simulink library "carnot"  (R2018b)
settings: Solver=VariableStepAuto  StartTime=0.0  StopTime=10.0  RelTol=1e-3
undefined symbols (not defined in the file or in its folder): A, A_earth, acol, Acol, ActPower1, ActPower2, ActPower3, Ad, Ad0, Ar, Au, Au0, Azimuth_Angle, B, Bd, Bd0, Br, Bu, Bu0, C, c1, c2, c3, c33, c4, c5, c6, CarnotCallbacks_Density, CarnotCallbacks_Enthalpy, CarnotCallbacks_Enthalpy2Temperature, CarnotCallbacks_Entropy, CarnotCallbacks_Evaporation_Enthalpy, CarnotCallbacks_GlobalMessageLevel, CarnotCallbacks_Grashof, CarnotCallbacks_Heat_Capacity, CarnotCallbacks_Kinematic_Viscosity, CarnotCallbacks_PMV_PPD, CarnotCallbacks_Prandtl, CarnotCallbacks_Saturation_Property, CarnotCallbacks_Saturation_Temperature, CarnotCallbacks_Saturation_Value_Water, CarnotCallbacks_Specific_Volume, CarnotCallbacks_Thermal_Conductivity, CarnotCallbacks_Vapour_Content, CarnotCallbacks_Vapour_Pressure, Cd, Cdl, Cr, Cu, Davies, Dd, DE_TRY2010_04_averageYear, delta_grd, density, DiameterLastPiece, dl, DPConstant, DPLinear, DPQuadratic, Dr ... (+59)
libraries: $bdroot x429, simulink x36, simulink_extras x12
(part 5 of 22)

== system carnot/Basic/Material_Properties ==
  AIV_WetBulbTemperature : Subsystem  mask(AIV to wet bulb temperature and relative humidity){}
      mask help:
      | Calculate  - the relative humidity of air (rH)
      |                  - and the wet bulb temperature of air (WBT)
      | from          - dry bulb air temperature (DBT)
      |                  - and mass of water per mass of air (x)
      | in AIV vector.
      |
      | DBT        [degree centigrade]
      | p              [Pa]
      | x              kg water / kg air
      |
      | rel_hum   [percent]
      | WBT       [degree centigrade] -> T_WBT is valid for T [-6..40°C]
      mask Help: web(fullfile(path_carnot('help'),'AIV_Wet_BulbTemperature.html'),'-helpbrowser')
  Density : Subsystem  LoadFcn=CarnotCallbacks_Density('LoadFcn');  InitFcn=load('THB.mat');  VariantControl=CarlibClassic  mask(density){INPUTARGUMENTS=state variables (classic), DEBUGLEVEL=DEBUGLEVEL, MAXTOTALWARNINGS=inf, MAXCONSECUTIVEWARNINGS=inf, WRITETOFILE=0, FILENAME='errors.txt'}
      mask prompts: INPUTARGUMENTS "Input arguments"; DEBUGLEVEL "Debug level"; MAXTOTALWARNINGS "maximum number of total warning"; MAXCONSECUTIVEWARNINGS "maximum number of consecutive warnings"; WRITETOFILE "write messages to file"; FILENAME "filename for error messages"
      mask help:
      | Calculates the fluid density  [kg/m³]. Calls the function "density" in the CARNOT library "carlib".
      | You may use the block "GlobalMessageLevel" in the Toolbox to handle the debugging messages.
      | FluidType        Remarks
      | 1: water          fluid mix is vapourcontent in the 2-phase region
      | 2: air              fluid mix is (kg water) / (kg dry air)
      | 3: cotton oil       -
      | 4: silicone oil     -
      | 5: water-glycol   fluid mix is volume partition [0..1] of propylen glycol
      | 6: Tyfocor LS     function only available in liquid phase
      | 7: Water Constant = 998.21 kg/m³ (water at 20°C)
      | 8: Air Constant   = 1.118 kg/m³ (air at 20°C)
      mask init:
      | %Inports
      | CarnotCallbacks_Density('CreateInports');
      | 
      | %global debug level
      | [DEBUGLEVEL, MAXTOTALWARNINGS, MAXCONSECUTIVEWARNINGS, WRITETOFILE, FILENAME] = CarnotCallbacks_Density('CheckDebugLevels', DEBUGLEVEL, MAXTOTALWARNINGS, MAXCONSECUTIVEWARNINGS, WRITETOFILE, FILENAME);
      mask Help: web(fullfile(path_carnot('help'),'density_mdl.html'),'-helpbrowser')
      mask TypeOptions INPUTARGUMENTS: state variables (classic) | THB | THV
      mask Callback INPUTARGUMENTS: CarnotCallbacks_Density('MaskVisibilities');
      mask TypeOptions DEBUGLEVEL: DEBUGLEVEL | INFOLEVEL | WARNINGLEVEL | ERRORLEVEL | FATALLEVEL | NOLEVEL
      mask DialogControl ParameterTabVar0 Prompt: Parameters
      mask DialogControl ParameterTabVar01 Prompt: Debugging
  Enthalpy : Subsystem  LoadFcn=CarnotCallbacks_Enthalpy('LoadFcn');  InitFcn=load('THB.mat');  VariantControl=CarlibClassic  mask(enthalpy){INPUTARGUMENTS=state variables (classic), DEBUGLEVEL=WARNINGLEVEL, MAXTOTALMESSAGES=inf, MAXCONSECUTIVEMESSAGES=inf, WRITETOFILE=0, FILENAME='errors.txt'}
      mask prompts: INPUTARGUMENTS "Input arguments"; DEBUGLEVEL "Debug level"; MAXTOTALMESSAGES "maximum number of total warning"; MAXCONSECUTIVEMESSAGES "maximum number of consecutive warnings"; WRITETOFILE "write messages to file"; FILENAME "filename for error messages"
      mask help:
      | Calculates the fluid specific enthalpy  [J/kg].
      | Calls the CARNOT library "carlib".
      | WORKS FOR WATER AND DRY AIR! Enthalpy for other fluids is cp*T.
      | FluidType        Remarks
      | 1: water          fluid mix is vapourcontent in the 2-phase region
      | 2: air              fluid mix is (kg water) / (kg dry air)
      | 3: cotton oil       -
      | 4: silicone oil     -
      | 5: water-glycol   fluid mix is volume partition [0..1] of propylen glycol
      | 6: Tyfocor LS     function only available in liquid phase
      | 7: Water Constant = 0.0 J/kg (water at 20°C)
      | 8: Air Constant   = 0.0 J/kg (air at 20°C)
      mask init:
      | %Inports
      | CarnotCallbacks_Enthalpy('CreateInports');
      | 
      | %global debug level
      | [DEBUGLEVEL, MAXTOTALMESSAGES, MAXCONSECUTIVEMESSAGES, WRITETOFILE, FILENAME] = CarnotCallbacks_Enthalpy('CheckDebugLevels', DEBUGLEVEL, MAXTOTALMESSAGES, MAXCONSECUTIVEMESSAGES, WRITETOFILE, FILENAME);
      mask Help: web(fullfile(path_carnot('help'),'enthalpy_mdl.html'),'-helpbrowser')
      mask TypeOptions INPUTARGUMENTS: state variables (classic) | THB | THV
      mask Callback INPUTARGUMENTS: CarnotCallbacks_Enthalpy('MaskVisibilities');
      mask TypeOptions DEBUGLEVEL: DEBUGLEVEL | INFOLEVEL | WARNINGLEVEL | ERRORLEVEL | FATALLEVEL | NOLEVEL
      mask DialogControl ParameterTabVar0 Prompt: Parameters
      mask DialogControl ParameterTabVar01 Prompt: Debugging
  Enthalpy2Temperature : Subsystem  LoadFcn=CarnotCallbacks_Enthalpy2Temperature('LoadFcn');  VariantControl=CarlibClassic  mask(Enthalpy to Temperature){DEBUGLEVEL=WARNINGLEVEL, MAXTOTALMESSAGES=inf, MAXCONSECUTIVEMESSAGES=inf, WRITETOFILE=0, FILENAME='errors.txt'}
      mask prompts: DEBUGLEVEL "Debug level"; MAXTOTALMESSAGES "maximum number of total warning"; MAXCONSECUTIVEMESSAGES "maximum number of consecutive warnings"; WRITETOFILE "write messages to file"; FILENAME "filename for error messages"
      mask help:
      | Calculates the temperature  [°C] from the fluid Enthalpy [J/kg].
      | Enthalpy may be a scalar or a vector. All other inputs must be scalar.
      | FluidType        Remarks
      | 1: water          fluid mix is vapourcontent in the 2-phase region
      | 2: air              fluid mix is (kg water) / (kg dry air)
      | 3: cotton oil       -
      | 4: silicone oil     -
      | 5: water-glycol   fluid mix is volume partition [0..1] of propylen glycol
      | 6: Tyfocor LS     function only available in liquid phase
      | 7: Water Constant - function not defined
      | 8: Air Constant - function not defined
      mask init:
      | %global debug level
      | [DEBUGLEVEL, MAXTOTALMESSAGES, MAXCONSECUTIVEMESSAGES, WRITETOFILE, FILENAME] = CarnotCallbacks_Enthalpy2Temperature('CheckDebugLevels', DEBUGLEVEL, MAXTOTALMESSAGES, MAXCONSECUTIVEMESSAGES, WRITETOFILE, FILENAME);
      mask Help: web(fullfile(path_carnot('help'),'enthalpy2temperature_mdl.html'),'-helpbrowser')
      mask TypeOptions DEBUGLEVEL: DEBUGLEVEL | INFOLEVEL | WARNINGLEVEL | ERRORLEVEL | FATALLEVEL | NOLEVEL
      mask DialogControl ParameterTabVar0 Prompt: Debugging
  Entropy : Subsystem  LoadFcn=CarnotCallbacks_Entropy('LoadFcn');  InitFcn=load('THB.mat');  VariantControl=CarlibClassic  mask(entropy){INPUTARGUMENTS=state variables (classic), DEBUGLEVEL=WARNINGLEVEL, MAXTOTALMESSAGES=inf, MAXCONSECUTIVEMESSAGES=inf, WRITETOFILE=0, FILENAME='errors.txt'}
      mask prompts: INPUTARGUMENTS "Input arguments"; DEBUGLEVEL "Debug level"; MAXTOTALMESSAGES "maximum number of total warning"; MAXCONSECUTIVEMESSAGES "maximum number of consecutive warnings"; WRITETOFILE "write messages to file"; FILENAME "filename for error messages"
      mask help:
      | The block calculates the entropy  [J/kgK] of the fluid.
      | The block calls the function "entropy" in the CARNOT library "carlib".
      | FluidType        Remarks
      | 1: water          fluid mix is vapourcontent in the 2-phase region
      | 2: air              fluid mix is (kg water) / (kg dry air)
      | 3: cotton oil       -
      | 4: silicone oil     -
      | 5: water-glycol   fluid mix is volume partition [0..1] of propylen glycol
      | 6: Tyfocor LS     function only available in liquid phase
      | 7: Water Constant = 0.0 J/K/kg
      | 8: Air Constant   = 0.0 J/K/kg
      mask init:
      | %Inports
      | CarnotCallbacks_Entropy('CreateInports');
      | 
      | %global debug level
      | [DEBUGLEVEL, MAXTOTALMESSAGES, MAXCONSECUTIVEMESSAGES, WRITETOFILE, FILENAME] = CarnotCallbacks_Entropy('CheckDebugLevels', DEBUGLEVEL, MAXTOTALMESSAGES, MAXCONSECUTIVEMESSAGES, WRITETOFILE, FILENAME);
      mask Help: web(fullfile(path_carnot('help'),'entropy.html'),'-helpbrowser')
      mask TypeOptions INPUTARGUMENTS: state variables (classic) | THB | THV
      mask Callback INPUTARGUMENTS: CarnotCallbacks_Entropy('MaskVisibilities');
      mask TypeOptions DEBUGLEVEL: DEBUGLEVEL | INFOLEVEL | WARNINGLEVEL | ERRORLEVEL | FATALLEVEL | NOLEVEL
      mask DialogControl ParameterTabVar0 Prompt: Parameters
      mask DialogControl ParameterTabVar01 Prompt: Debugging
  Evaporation_Enthalpy : Subsystem  LoadFcn=CarnotCallbacks_Evaporation_Enthalpy('LoadFcn');  InitFcn=load('THB.mat');  VariantControl=CarlibClassic  mask(entropy){INPUTARGUMENTS=state variables (classic), DEBUGLEVEL=WARNINGLEVEL, MAXTOTALMESSAGES=inf, MAXCONSECUTIVEMESSAGES=inf, WRITETOFILE=0, FILENAME='errors.txt'}
      mask prompts: INPUTARGUMENTS "Input arguments"; DEBUGLEVEL "Debug level"; MAXTOTALMESSAGES "maximum number of total warning"; MAXCONSECUTIVEMESSAGES "maximum number of consecutive warnings"; WRITETOFILE "write messages to file"; FILENAME "filename for error messages"
      mask help:
      | The block calculates the evaporation enthalpy [J/kgK] of water.
      | The block uses the material properties functions in carlib.
      | FluidType  material           remarks on fluid mix
      | 1           water              vapourcontent in the 2-phase region
      | all others: function not defined
      mask init:
      | %Inports
      | CarnotCallbacks_Evaporation_Enthalpy('CreateInports');
      | 
      | %global debug level
      | [DEBUGLEVEL, MAXTOTALMESSAGES, MAXCONSECUTIVEMESSAGES, WRITETOFILE, FILENAME] = CarnotCallbacks_Evaporation_Enthalpy('CheckDebugLevels', DEBUGLEVEL, MAXTOTALMESSAGES, MAXCONSECUTIVEMESSAGES, WRITETOFILE, FILENAME);
      mask Help: web(fullfile(path_carnot('help'),'evaporation_enthalpy_mdl.html'),'-helpbrowser')
      mask TypeOptions INPUTARGUMENTS: state variables (classic) | THB | THV
      mask Callback INPUTARGUMENTS: CarnotCallbacks_Evaporation_Enthalpy('MaskVisibilities');
      mask TypeOptions DEBUGLEVEL: DEBUGLEVEL | INFOLEVEL | WARNINGLEVEL | ERRORLEVEL | FATALLEVEL | NOLEVEL
      mask DialogControl ParameterTabVar0 Prompt: Parameters
      mask DialogControl ParameterTabVar01 Prompt: Debugging
  Heat_Capacity : Subsystem  LoadFcn=CarnotCallbacks_Heat_Capacity('LoadFcn');  InitFcn=load('THB.mat');  VariantControl=CarlibClassic  mask(heat capacity){INPUTARGUMENTS=state variables (classic), DEBUGLEVEL=DEBUGLEVEL, MAXTOTALWARNINGS=inf, MAXCONSECUTIVEWARNINGS=inf, WRITETOFILE=0, FILENAME='errors.txt'}
      mask prompts: INPUTARGUMENTS "Input arguments"; DEBUGLEVEL "Debug level"; MAXTOTALWARNINGS "maximum number of total warning"; MAXCONSECUTIVEWARNINGS "maximum number of consecutive warnings"; WRITETOFILE "write messages to file"; FILENAME "filename for error messages"
      mask help:
      | Calculates the  heat_capacity of fluids [J/(kg*K)]. Calls calls the function "heat_capacity" in the CARNOT library "carlib".
      | You may use the block "GlobalMessageLevel" in the Toolbox to handle the debugging messages.
      | FluidType        Remarks
      | 1: water          fluid mix is vapourcontent in the 2-phase region
      | 2: air              fluid mix is (kg water) / (kg dry air)
      | 3: cotton oil       -
      | 4: silicone oil     -
      | 5: water-glycol   fluid mix is volume partition [0..1] of propylen glycol
      | 6: Tyfocor LS     function only available in liquid phase
      | 7: Water Constant = 4181.0 J/kg/K (water at 20°C)
      | 8: Air Constant   = 1007.0 J/kg/K (air at 20°C)
      mask init:
      | %Inports
      | CarnotCallbacks_Heat_Capacity('CreateInports');
      | 
      | %global debug level
      | [DEBUGLEVEL, MAXTOTALWARNINGS, MAXCONSECUTIVEWARNINGS, WRITETOFILE, FILENAME] = CarnotCallbacks_Heat_Capacity('CheckDebugLevels', DEBUGLEVEL, MAXTOTALWARNINGS, MAXCONSECUTIVEWARNINGS, WRITETOFILE, FILENAME);
      mask Help: web(fullfile(path_carnot('help'),'heat_capacity_mdl.html'),'-helpbrowser')
      mask TypeOptions INPUTARGUMENTS: state variables (classic) | THB | THV
      mask Callback INPUTARGUMENTS: CarnotCallbacks_Heat_Capacity('MaskVisibilities');
      mask TypeOptions DEBUGLEVEL: DEBUGLEVEL | INFOLEVEL | WARNINGLEVEL | ERRORLEVEL | FATALLEVEL | NOLEVEL
      mask DialogControl ParameterTabVar0 Prompt: Parameters
      mask DialogControl ParameterTabVar01 Prompt: Debugging
  Input_Air : Subsystem  mask(Input_Air){T=20, p=1e5, x=0.005}
      mask prompts: T "temperature (scalar or vector) [°C]"; p "pressure [Pa]"; x "absolute humidity of moist air [kg water/kg dry air]"
      mask help:
      | Input block for the material "Air"
      |
      | The relevant inputs for the calculation of the block can be specified as parameter in the mask
      mask Help: web(fullfile(path_carnot('help'),'input_material.html'),'-helpbrowser')
  Input_Cotton_Oil : Subsystem  mask(Input_Cotton_Oil){T=20, p=1e5}
      mask prompts: T "temperature (scalar or vector) [°C]"; p "pressure [Pa]"
      mask help: Input block for the material "Cotton Oil". The relevant inputs for the calculation of the block can be specified as parameter in the mask
      mask Help: web(fullfile(path_carnot('help'),'input_material.html'),'-helpbrowser')
  Input_Fluid : Subsystem  mask(Input_Fluid){fluid=Water, T=[10:10:50], p=1e5, x=0.005}
      mask prompts: fluid "Fluid type"; T "temperature (scalar or vector) [°C]"; p "pressure [Pa]"; x "Fluid Mix"
      mask help:
      | FLUID            FLUID MIX
      | water          vapourcontent in the 2-phase region
      | air               (kg water) / (kg dry air)
      | cotton oil       -
      | silicone oil     -
      | water-glycol   volume partition [0..1] of propylen glycol
      mask Help: web(fullfile(path_carnot('help'),'input_material.html'),'-helpbrowser')
      mask TypeOptions fluid: Water | Air | Cotton Oil | Silicone Oil | Water-Glycol Mix | Tyfocor LS | Water (Constant 20°C) | Air (dry+ constant 20°C)
  Input_Silicon_Oil : Subsystem  mask(Input_Silicon_Oil){T=20, p=1e5}
      mask prompts: T "temperature (scalar or vector) [°C]"; p "pressure [Pa]"
      mask help: Input block for the material "Silicon_Oil". The relevant inputs for the calculation of the block can be specified as parameter in the mask
      mask Help: web(fullfile(path_carnot('help'),'input_material.html'),'-helpbrowser')
  Input_Tyfocor_LS : Subsystem  mask(Input_Tyfocor_LS){T=20, p=1e5}
      mask prompts: T "temperature (scalar or vector) [°C]"; p "pressure [Pa]"
      mask help:
      | Input block for the material "Tyfocor_LS". The relevant inputs for the calculation of the block can be specified as parameter in the mask.
      | Tyfocor is a registered trademark of Tyforop Chemie, Hamburg (Germany).
      mask Help: web(fullfile(path_carnot('help'),'input_material.html'),'-helpbrowser')
  Input_Water : Subsystem  mask(Input_Water){T=20, p=2e6, xd=0}
      mask prompts: T "temperature (scalar or vector) [°C]"; p "pressure [Pa]"; xd "vapour content of the water [0..1]"
      mask help:
      | Input block for the material "Water"
      |
      | The relevant inputs for the calculation of the block can be specified as parameter in the mask
      mask Help: web(fullfile(path_carnot('help'),'input_material.html'),'-helpbrowser')
  Input_Water_Glycol : Subsystem  mask(input_water_glycol){T=20, p=1e5, g=0.4}
      mask prompts: T "temperature (scalar or vector) [°C]"; p "pressure [Pa]"; g "volume content of glycol [0..1]"
      mask help: Sets all values for the water - propylen-glycol mixtures.
      mask Help: web(fullfile(path_carnot('help'),'input_material.html'),'-helpbrowser')
  Kinematic_Viscosity : Subsystem  LoadFcn=CarnotCallbacks_Kinematic_Viscosity('LoadFcn');  InitFcn=load('THB.mat');  VariantControl=CarlibClassic  mask(kinematic viscosity){INPUTARGUMENTS=state variables (classic), DEBUGLEVEL=WARNINGLEVEL, MAXTOTALMESSAGES=inf, MAXCONSECUTIVEMESSAGES=inf, WRITETOFILE=0, FILENAME='errors.txt'}
      mask prompts: INPUTARGUMENTS "Input arguments"; DEBUGLEVEL "Debug level"; MAXTOTALMESSAGES "maximum number of total warning"; MAXCONSECUTIVEMESSAGES "maximum number of consecutive warnings"; WRITETOFILE "write messages to file"; FILENAME "filename for error messages"
      mask help:
      | Calculates the kinematic viscosity of fluids [m²/s].
      | Calls the function "viscosity" in the CARNOT library "carlib".
      | FluidType        Remarks
      | 1: water          fluid mix is vapourcontent in the 2-phase region
      | 2: air              fluid mix is (kg water) / (kg dry air)
      | 3: cotton oil       -
      | 4: silicone oil     -
      | 5: water-glycol   fluid mix is volume partition [0..1] of propylen glycol
      | 6: Tyfocor LS     function only available in liquid phase
      | 7: Water Constant = 1.004e-6 m²/s (water at 20°C)
      | 8: Air Constant   = 15.35e-6 m²/s (air at 20°C)
      mask init:
      | %Inports
      | CarnotCallbacks_Kinematic_Viscosity('CreateInports');
      | 
      | %global debug level
      | [DEBUGLEVEL, MAXTOTALMESSAGES, MAXCONSECUTIVEMESSAGES, WRITETOFILE, FILENAME] = CarnotCallbacks_Kinematic_Viscosity('CheckDebugLevels', DEBUGLEVEL, MAXTOTALMESSAGES, MAXCONSECUTIVEMESSAGES, WRITETOFILE, FILENAME);
      mask Help: web(fullfile(path_carnot('help'),'kinematic_viscosity_mdl.html'),'-helpbrowser')
      mask TypeOptions INPUTARGUMENTS: state variables (classic) | THB | THV
      mask Callback INPUTARGUMENTS: CarnotCallbacks_Kinematic_Viscosity('MaskVisibilities');
      mask TypeOptions DEBUGLEVEL: DEBUGLEVEL | INFOLEVEL | WARNINGLEVEL | ERRORLEVEL | FATALLEVEL | NOLEVEL
      mask DialogControl ParameterTabVar0 Prompt: Parameters
      mask DialogControl ParameterTabVar01 Prompt: Debugging
  PhaseCheck : Subsystem  mask(phasecheck){}
      mask help: Checks whether fluid is still in the correct phase, for example if water is not steam or ice. Simulation is stopped for inconstistent phase.
      mask Help: web(fullfile(path_carnot('help'),'PhaseCheck.html'),'-helpbrowser')
  RelHum2x : Subsystem  mask(relative humidity to x){}
      mask help:
      | Calculate the mass of water per mass of air (x)
      | from the relative humidity of air.
      |
      | T             [degree centigrade]
      | p             [Pa]
      | rel_hum   [percent]
      | x              kg water / kg air
      mask Help: web(fullfile(path_carnot('help'),'RelHum2x.html'),'-helpbrowser')
  Saturation_Property : Subsystem  LoadFcn=CarnotCallbacks_Saturation_Property('LoadFcn');  InitFcn=load('THB.mat');  VariantControl=CarlibClassic  mask(saturation property){INPUTARGUMENTS=state variables (classic), PROPERTY=density, FLUIDPHASE=liquid, DEBUGLEVEL=WARNINGLEVEL, MAXTOTALMESSAGES=inf, MAXCONSECUTIVEMESSAGES=inf, WRITETOFILE=0, FILENAME='errors.txt'}
      mask prompts: INPUTARGUMENTS "Input arguments"; FLUIDPHASE "fluid phase"; DEBUGLEVEL "Debug level"; MAXTOTALMESSAGES "maximum number of total warning"; MAXCONSECUTIVEMESSAGES "maximum number of consecutive warnings"; WRITETOFILE "write messages to file"; FILENAME "filename for error messages"
      mask help:
      | The block calculates the saturation value of water by the value of a specified property. Calls the function "saturationproperty" in the CARNOT library "Carlib".
      |
      | PROPERTY            UNIT
      | density                     kg/m³
      | heat capacity           J/kgK
      | heat conductivity     W/mK
      | kinematic viscosity   m²/s
      | enthalpy                   J/kg
      | entropy                     J/kgK
      | prandtl                      --
      | specific volume        m³/kg
      mask init:
      | %Inports
      | CarnotCallbacks_Saturation_Property('CreateInports');
      | 
      | %global debug level
      | [DEBUGLEVEL, MAXTOTALMESSAGES, MAXCONSECUTIVEMESSAGES, WRITETOFILE, FILENAME] = CarnotCallbacks_Saturation_Property('CheckDebugLevels', DEBUGLEVEL, MAXTOTALMESSAGES, MAXCONSECUTIVEMESSAGES, WRITETOFILE, FILENAME);
      mask Help: web(fullfile(path_carnot('help'),'saturationproperty.html'),'-helpbrowser')
      mask TypeOptions INPUTARGUMENTS: state variables (classic) | THB | THV
      mask Callback INPUTARGUMENTS: CarnotCallbacks_Saturation_Property('MaskVisibilities');
      mask TypeOptions PROPERTY: density | heat capacity | heat conductivity | kinematic viscosity | enthalpy | entropy | prandtl | specific volume
      mask TypeOptions FLUIDPHASE: vaporous | liquid | solid
      mask TypeOptions DEBUGLEVEL: DEBUGLEVEL | INFOLEVEL | WARNINGLEVEL | ERRORLEVEL | FATALLEVEL | NOLEVEL
      mask DialogControl ParameterTabVar0 Prompt: Parameters
      mask DialogControl ParameterTabVar01 Prompt: Debugging
  Saturation_Temperature : Subsystem  LoadFcn=CarnotCallbacks_Saturation_Temperature('LoadFcn');  InitFcn=load('THB.mat');  VariantControl=CarlibClassic  mask(Saturation Temperature){INPUTARGUMENTS=state variables (classic), DEBUGLEVEL=WARNINGLEVEL, MAXTOTALMESSAGES=inf, MAXCONSECUTIVEMESSAGES=inf, WRITETOFILE=0, FILENAME='errors.txt'}
      mask prompts: INPUTARGUMENTS "Input arguments"; DEBUGLEVEL "Debug level"; MAXTOTALMESSAGES "maximum number of total warning"; MAXCONSECUTIVEMESSAGES "maximum number of consecutive warnings"; WRITETOFILE "write messages to file"; FILENAME "filename for error messages"
      mask help:
      | Calculates the saturationtemperature in °C
      | Fluid Type 1 - water or water mixtures: temperature of saturated steam as a function of pressure.
      | Fluid Type 2 - moist air: dew point temperature of the moist air as a function of water content. Input fluid mix (kg water / kg air) may be a vector.
      mask init:
      | %Inports
      | CarnotCallbacks_Saturation_Temperature('CreateInports');
      | 
      | %global debug level
      | [DEBUGLEVEL, MAXTOTALMESSAGES, MAXCONSECUTIVEMESSAGES, WRITETOFILE, FILENAME] = CarnotCallbacks_Saturation_Temperature('CheckDebugLevels', DEBUGLEVEL, MAXTOTALMESSAGES, MAXCONSECUTIVEMESSAGES, WRITETOFILE, FILENAME);
      mask Help: web(fullfile(path_carnot('help'),'Saturation_Temperature.html'),'-helpbrowser')
      mask TypeOptions INPUTARGUMENTS: state variables (classic) | THB | THV
      mask Callback INPUTARGUMENTS: CarnotCallbacks_Saturation_Temperature('MaskVisibilities');
      mask TypeOptions DEBUGLEVEL: DEBUGLEVEL | INFOLEVEL | WARNINGLEVEL | ERRORLEVEL | FATALLEVEL | NOLEVEL
      mask DialogControl ParameterTabVar0 Prompt: Parameters
      mask DialogControl ParameterTabVar01 Prompt: Debugging
  Saturation_Value_Water : Subsystem  LoadFcn=CarnotCallbacks_Saturation_Value_Water('LoadFcn');  InitFcn=load('THB.mat');  VariantControl=CarlibClassic  mask(saturation value water){INPUTARGUMENTS=state variables (classic), DEBUGLEVEL=WARNINGLEVEL, MAXTOTALMESSAGES=inf, MAXCONSECUTIVEMESSAGES=inf, WRITETOFILE=0, FILENAME='errors.txt'}
      mask prompts: INPUTARGUMENTS "Input arguments"; DEBUGLEVEL "Debug level"; MAXTOTALMESSAGES "maximum number of total warning"; MAXCONSECUTIVEMESSAGES "maximum number of consecutive warnings"; WRITETOFILE "write messages to file"; FILENAME "filename for error messages"
      mask help:
      | Calculates the saturation value of fluid by the value of a specified property.
      | Temperature may be a scalar or vector, all other inputs must be scalar.
      | property-ID        property                       unit
      | 1                       density                         [kg/m³]
      | 2                       heat capacity               [J/kgK]
      | 3                       heat conductivity         [W/mK]
      | 4                       kinematic viscosity       [m²/s]
      | 5                       enthalpy                       [J/kg]
      | 6                       entropy                         [J/kgK]
      | 7                       prandtl                          [-]
      | 8                       specific volume            [m³/kg]
      | not defined for this function
      | 9                       evaporation  enthalpy  [J/kg]
      | 10                     vapourpressure            [Pa]
      | 11                     saturationtemperatur    [°C]
      mask init:
      | %Inports
      | CarnotCallbacks_Saturation_Value_Water('CreateInports');
      | 
      | %global debug level
      | [DEBUGLEVEL, MAXTOTALMESSAGES, MAXCONSECUTIVEMESSAGES, WRITETOFILE, FILENAME] = CarnotCallbacks_Saturation_Value_Water('CheckDebugLevels', DEBUGLEVEL, MAXTOTALMESSAGES, MAXCONSECUTIVEMESSAGES, WRITETOFILE, FILENAME);
      mask Help: web(fullfile(path_carnot('help'),'saturationvalue_water.html'),'-helpbrowser')
      mask TypeOptions INPUTARGUMENTS: state variables (classic) | THB | THV
      mask Callback INPUTARGUMENTS: CarnotCallbacks_Saturation_Value_Water('MaskVisibilities');
      mask TypeOptions DEBUGLEVEL: DEBUGLEVEL | INFOLEVEL | WARNINGLEVEL | ERRORLEVEL | FATALLEVEL | NOLEVEL
      mask DialogControl ParameterTabVar0 Prompt: Parameters
      mask DialogControl ParameterTabVar01 Prompt: Debugging
  Specific_Volume : Subsystem  LoadFcn=CarnotCallbacks_Specific_Volume('LoadFcn');  InitFcn=load('THB.mat');  VariantControl=CarlibClassic  mask(specific volume){INPUTARGUMENTS=state variables (classic), DEBUGLEVEL=DEBUGLEVEL, MAXTOTALWARNINGS=inf, MAXCONSECUTIVEWARNINGS=inf, WRITETOFILE=0, FILENAME='errors.txt'}
      mask prompts: INPUTARGUMENTS "Input arguments"; DEBUGLEVEL "Debug level"; MAXTOTALWARNINGS "maximum number of total warning"; MAXCONSECUTIVEWARNINGS "maximum number of consecutive warnings"; WRITETOFILE "write messages to file"; FILENAME "filename for error messages"
      mask help:
      | Calculates the specific volume of fluids [m³/kg]. Calls the function "specific_volume" in the CARNOT library "Carlib".
      | You may use the block "GlobalMessageLevel" in the Toolbox to handle the debugging messages.
      | FluidType        Remarks
      | 1: water          fluid mix is vapourcontent in the 2-phase region
      | 2: air              fluid mix is (kg water) / (kg dry air)
      | 3: cotton oil       -
      | 4: silicone oil     -
      | 5: water-glycol   fluid mix is volume partition [0..1] of propylen glycol
      | 6: Tyfocor LS     function only available in liquid phase
      | 7: Water Constant = 1.0 / 998.21 m³/kg (water at 20°C)
      | 8: Air Constant   = 1.0 / 1.118 m³/kg (air at 20°C)
      mask init:
      | %Inports
      | CarnotCallbacks_Specific_Volume('CreateInports');
      | 
      | %global debug level
      | [DEBUGLEVEL, MAXTOTALWARNINGS, MAXCONSECUTIVEWARNINGS, WRITETOFILE, FILENAME] = CarnotCallbacks_Specific_Volume('CheckDebugLevels', DEBUGLEVEL, MAXTOTALWARNINGS, MAXCONSECUTIVEWARNINGS, WRITETOFILE, FILENAME);
      mask Help: web(fullfile(path_carnot('help'),'Specific_Volume_mdl.html'),'-helpbrowser')
      mask TypeOptions INPUTARGUMENTS: state variables (classic) | THB | THV
      mask Callback INPUTARGUMENTS: CarnotCallbacks_Specific_Volume('MaskVisibilities');
      mask TypeOptions DEBUGLEVEL: DEBUGLEVEL | INFOLEVEL | WARNINGLEVEL | ERRORLEVEL | FATALLEVEL | NOLEVEL
      mask DialogControl ParameterTabVar0 Prompt: Parameters
      mask DialogControl ParameterTabVar01 Prompt: Debugging
  THB_WetBulbTemperature : Subsystem  mask(THB to wet bulb temperature and relative humidity){}
      mask help:
      | Calculate  - the relative humidity of air (rH)
      |                  - and the wet bulb temperature of air (WBT)
      | from          - dry bulb air temperature (DBT)
      |                  - and mass of water per mass of air (x)
      | in THV vector.
      |
      | DBT        [degree centigrade]
      | p              [Pa]
      | x              kg water / kg air
      |
      | rel_hum   [percent]
      | WBT       [degree centigrade] -> T_WBT is valid for T [-6..40°C]
      mask Help: web(fullfile(path_carnot('help'),'THB_Wet_BulbTemperature.html'),'-helpbrowser')
  Temperature_Conductivity : Subsystem  LoadFcn=CarnotCallbacks_Thermal_Conductivity('LoadFcn');  InitFcn=load('THB.mat');  VariantControl=CarlibClassic  mask(temperature conductivity){INPUTARGUMENTS=state variables (classic), DEBUGLEVEL=WARNINGLEVEL, MAXTOTALMESSAGES=inf, MAXCONSECUTIVEMESSAGES=inf, WRITETOFILE=0, FILENAME='errors.txt'}
      mask prompts: INPUTARGUMENTS "Input arguments"; DEBUGLEVEL "Debug level"; MAXTOTALMESSAGES "maximum number of total warning"; MAXCONSECUTIVEMESSAGES "maximum number of consecutive warnings"; WRITETOFILE "write messages to file"; FILENAME "filename for error messages"
      mask help:
      | Calclulates the temperature conductivity of fluids in [m²/s]. Calls the function "cond" in the CARNOT library "carlib".
      | Temperature input may be a vector with several elements.
      | You may use the block "GlobalMessageLevel" in the Toolbox to handle the debugging messages.
      | FluidType        Remarks
      | 1: water          fluid mix is vapourcontent in the 2-phase region
      | 2: air              fluid mix is (kg water) / (kg dry air)
      | 3: cotton oil       -
      | 4: silicone oil     -
      | 5: water-glycol   fluid mix is volume partition [0..1] of propylen glycol
      | 6: Tyfocor LS     function only available in liquid phase
      | 7: Water Constant =  0.5984 W/m/K (water at 20°C)
      | 8: Air Constant   =  0.02569 W/m/K (air at 20°C)
      mask init:
      | %Inports
      | CarnotCallbacks_Thermal_Conductivity('CreateInports');
      | 
      | %global debug level
      | [DEBUGLEVEL, MAXTOTALMESSAGES, MAXCONSECUTIVEMESSAGES, WRITETOFILE, FILENAME] = CarnotCallbacks_Thermal_Conductivity('CheckDebugLevels', DEBUGLEVEL, MAXTOTALMESSAGES, MAXCONSECUTIVEMESSAGES, WRITETOFILE, FILENAME);
      mask Help: web(fullfile(path_carnot('help'),'Temperature_Conductivity_mdl.html'),'-helpbrowser')
      mask TypeOptions INPUTARGUMENTS: state variables (classic) | THB | THV
      mask Callback INPUTARGUMENTS: CarnotCallbacks_Thermal_Conductivity('MaskVisibilities');
      mask TypeOptions DEBUGLEVEL: DEBUGLEVEL | INFOLEVEL | WARNINGLEVEL | ERRORLEVEL | FATALLEVEL | NOLEVEL
      mask DialogControl ParameterTabVar0 Prompt: Parameters
      mask DialogControl ParameterTabVar01 Prompt: Debugging
  Thermal_Conductivity : Subsystem  LoadFcn=CarnotCallbacks_Thermal_Conductivity('LoadFcn');  InitFcn=load('THB.mat');  VariantControl=CarlibClassic  mask(thermal conductivity){INPUTARGUMENTS=state variables (classic), DEBUGLEVEL=WARNINGLEVEL, MAXTOTALMESSAGES=inf, MAXCONSECUTIVEMESSAGES=inf, WRITETOFILE=0, FILENAME='errors.txt'}
      mask prompts: INPUTARGUMENTS "Input arguments"; DEBUGLEVEL "Debug level"; MAXTOTALMESSAGES "maximum number of total warning"; MAXCONSECUTIVEMESSAGES "maximum number of consecutive warnings"; WRITETOFILE "write messages to file"; FILENAME "filename for error messages"
      mask help:
      | Calclulates the thermal conductivity of fluids in [W/(m*K)]. Calls the function "cond" in the CARNOT library "carlib".
      | Temperature input may be a vector with several elements.
      | You may use the block "GlobalMessageLevel" in the Toolbox to handle the debugging messages.
      | FluidType        Remarks
      | 1: water          fluid mix is vapourcontent in the 2-phase region
      | 2: air              fluid mix is (kg water) / (kg dry air)
      | 3: cotton oil       -
      | 4: silicone oil     -
      | 5: water-glycol   fluid mix is volume partition [0..1] of propylen glycol
      | 6: Tyfocor LS     function only available in liquid phase
      | 7: Water Constant =  0.5984 W/m/K (water at 20°C)
      | 8: Air Constant   =  0.02569 W/m/K (air at 20°C)
      mask init: same as carnot/Basic/Material_Properties/Temperature_Conductivity
      mask Help: web(fullfile(path_carnot('help'),'thermal_conductivity_mdl.html'),'-helpbrowser')
      mask TypeOptions INPUTARGUMENTS: state variables (classic) | THB | THV
      mask Callback INPUTARGUMENTS: CarnotCallbacks_Thermal_Conductivity('MaskVisibilities');
      mask TypeOptions DEBUGLEVEL: DEBUGLEVEL | INFOLEVEL | WARNINGLEVEL | ERRORLEVEL | FATALLEVEL | NOLEVEL
      mask DialogControl ParameterTabVar0 Prompt: Parameters
      mask DialogControl ParameterTabVar01 Prompt: Debugging
  Vapour_Content : Subsystem  LoadFcn=CarnotCallbacks_Vapour_Content('LoadFcn');  InitFcn=load('THB.mat');  VariantControl=CarlibClassic  mask(vapourcontent){INPUTARGUMENTS=state variables (classic), PROPERTYTYPE=density, DEBUGLEVEL=WARNINGLEVEL, MAXTOTALMESSAGES=inf, MAXCONSECUTIVEMESSAGES=inf, WRITETOFILE=0, FILENAME='errors.txt'}
      mask prompts: INPUTARGUMENTS "Input arguments"; PROPERTYTYPE "property type"; DEBUGLEVEL "Debug level"; MAXTOTALMESSAGES "maximum number of total warning"; MAXCONSECUTIVEMESSAGES "maximum number of consecutive warnings"; WRITETOFILE "write messages to file"; FILENAME "filename for error messages"
      mask help:
      | The block calculates the (water-)vapour content of water or water-glycol mixture by the value of a specified property. The block calls the function "vapourcontent" in the CARNOT library "Carlib".
      | Temperature and the "Value" may be a scalar or vector, all other inputs must be scalar (length of "temperature" and "value" must be same).
      | You may use the block "GlobalMessageLevel" in the Toolbox to handle the debugging messages.
      | Definition of property-types
      | property                    unit
      |  density                     [kg/m³]
      |  heat capacity           [J/kgK]
      |  heat conductivity     [W/mK]
      |  kinematic viscosity   [m²/s]
      |  enthalpy                   [J/kg]
      |  entropy                     [J/kgK]
      |  prandtl                      [-]
      |  specific volume        [m³/kg]
      mask init:
      | %Inports
      | CarnotCallbacks_Vapour_Content('CreateInports');
      | 
      | %global debug level
      | [DEBUGLEVEL, MAXTOTALMESSAGES, MAXCONSECUTIVEMESSAGES, WRITETOFILE, FILENAME] = CarnotCallbacks_Vapour_Content('CheckDebugLevels', DEBUGLEVEL, MAXTOTALMESSAGES, MAXCONSECUTIVEMESSAGES, WRITETOFILE, FILENAME);
      mask Help: web(fullfile(path_carnot('help'),'vapour_content.html'),'-helpbrowser')
      mask TypeOptions INPUTARGUMENTS: state variables (classic) | THB | THV
      mask Callback INPUTARGUMENTS: CarnotCallbacks_Vapour_Content('MaskVisibilities');
      mask TypeOptions PROPERTYTYPE: density | heat capacity | heat conductivity | kinematic viscosity | enthalpy | entropy | prandtl | specific volume
      mask TypeOptions DEBUGLEVEL: DEBUGLEVEL | INFOLEVEL | WARNINGLEVEL | ERRORLEVEL | FATALLEVEL | NOLEVEL
      mask DialogControl ParameterTabVar0 Prompt: Parameters
      mask DialogControl ParameterTabVar01 Prompt: Debugging
  Vapour_Pressure : Subsystem  LoadFcn=CarnotCallbacks_Vapour_Pressure('LoadFcn');  InitFcn=load('THB.mat');  VariantControl=CarlibClassic  mask(vapourpressure){INPUTARGUMENTS=state variables (classic), DEBUGLEVEL=WARNINGLEVEL, MAXTOTALMESSAGES=inf, MAXCONSECUTIVEMESSAGES=inf, WRITETOFILE=0, FILENAME='errors.txt'}
      mask prompts: INPUTARGUMENTS "Input arguments"; DEBUGLEVEL "Debug level"; MAXTOTALMESSAGES "maximum number of total warning"; MAXCONSECUTIVEMESSAGES "maximum number of consecutive warnings"; WRITETOFILE "write messages to file"; FILENAME "filename for error messages"
      mask help:
      | Calculates the vapour pressure of fluids [Pa]. Calls the function "vapourpressure" in the CARNOT library "Carlib".
      | You may use the block "GlobalMessageLevel" in the Toolbox to handle the debugging messages.
      | FluidType        Remarks
      | 1: water          fluid mix is vapourcontent in the 2-phase region
      | 2: air              fluid mix is (kg water) / (kg dry air)
      | 3: cotton oil       function not defined
      | 4: silicone oil     function not defined
      | 5: water-glycol   fluid mix is volume partition [0..1] of propylen glycol
      | 6: Tyfocor LS     function only available in liquid phase
      | 7: Water Constant function not defined
      | 8: Air Constant   function not defined
      mask init:
      | %Inports
      | CarnotCallbacks_Vapour_Pressure('CreateInports');
      | 
      | %global debug level
      | [DEBUGLEVEL, MAXTOTALMESSAGES, MAXCONSECUTIVEMESSAGES, WRITETOFILE, FILENAME] = CarnotCallbacks_Vapour_Pressure('CheckDebugLevels', DEBUGLEVEL, MAXTOTALMESSAGES, MAXCONSECUTIVEMESSAGES, WRITETOFILE, FILENAME);
      mask Help: web(fullfile(path_carnot('help'),'vapourpressure.html'),'-helpbrowser')
      mask TypeOptions INPUTARGUMENTS: state variables (classic) | THB | THV
      mask Callback INPUTARGUMENTS: CarnotCallbacks_Vapour_Pressure('MaskVisibilities');
      mask TypeOptions DEBUGLEVEL: DEBUGLEVEL | INFOLEVEL | WARNINGLEVEL | ERRORLEVEL | FATALLEVEL | NOLEVEL
      mask DialogControl ParameterTabVar0 Prompt: Parameters
      mask DialogControl ParameterTabVar01 Prompt: Debugging
  x2RelHum : Subsystem  mask(x to relative humidity){}
      mask help:
      | Calculate  the relative humidity of air
      | from the mass of water per mass of air (x).
      |
      | T             [°C]
      | p             [Pa]
      | rel_hum   [percent]
      | x              kg water / kg dry air
      mask Help: web(fullfile(path_carnot('help'),'x2rel_hum.html'),'-helpbrowser')

== system carnot/Basic/Pressure_Drop ==
  Pressure_Drop : Subsystem  mask(pressure drop){}
      mask help:
      | Pressure drop according to input values of con, lin and qua:
      | dp = con + lin*mdot + qua*mdot²
      | The coefficients are also added to the correponding THB elements.
      mask Help: web(fullfile(path_carnot('help'),'Pressure_Drop.html'),'-helpbrowser')
  Pressure_Drop_Ceta : Subsystem  mask(fixed pressure drop){con=101, lin=202, qua=303}
      mask prompts: con "c : constant (static) pressure drop in Pa"; lin "l : linear pressure drop Pa/(kg/s)"; qua "q : quadratic pressure drop Pa/(kg/s)²"
      mask help:
      | Calculates the pressure drop from a pressure drop coefficient ceta:
      | dp = ceta * density/2 * velocity²
      | Calculation is done for ID > 10000 (dp = f(l, q), c is neglected) and ID > 20000 (dp = f(c,l,q)).
      | Applied directly to the THB bus.
      mask Help: web(fullfile(path_carnot('help'),'Pressure_Drop_Ceta.html'),'-helpbrowser')
  Pressure_Drop_Collector : Subsystem  mask(Pressure Drop Collector){len=1, lin=100, qua=100}
      mask prompts: len "Length of collector in m"; lin "l : linear pressure drop Pa/(kg/s)"; qua "q : quadratic pressure drop Pa/(kg/s)²"
      mask help:
      | Calculates the pressure drop according to constant values of con, lin and qua:
      | dp_dyn = c + l*mdot + q*mdot²
      | Static height is taken in account via the collector inclination, the length and the temperatures:
      | dp_stat = density * grav * height
      | Total pressure is dp = dp_dyn + dpstat
      mask Help: web(fullfile(path_carnot('help'),'Pressure_Drop_Collector.html'),'-helpbrowser')
      mask TypeOptions len: Gain/Gain
      mask TypeOptions lin: Pressure_Drop_Fix/lin
      mask TypeOptions qua: Pressure_Drop_Fix/qua
  Pressure_Drop_Fix : Subsystem  mask(fixed pressure drop){con=101, lin=202, qua=303}
      mask prompts: con "c : constant (static) pressure drop in Pa"; lin "l : linear pressure drop Pa/(kg/s)"; qua "q : quadratic pressure drop Pa/(kg/s)²"
      mask help:
      | Constant parameters for pressure drop in a flow.
      | dp = c + l*mdot + q*mdot²
      | Calculation is done for ID > 10000 (dp = f(l, q), c is neglected) and ID > 20000 (dp = f(c,l,q)).
      | Applied directly to the THB bus.
      mask Help: web(fullfile(path_carnot('help'),'Pressure_Drop_Fix.html'),'-helpbrowser')
  Pressure_Drop_PipeTheory : Subsystem  mask(theoretical pressure drop of a pipe){dia=0.02, len=1, rough=0.04, nbend=1}
      mask prompts: dia "Diameter in m"; len "Length of pipe in m"; rough "Roughness of pipe in m"; nbend "Number of 90° bends"
      mask help: Calculates the pressure drop in a pipe according to a theoretical model.
      mask Help: web(fullfile(path_carnot('help'),'Pressure_Drop_PipeTheory.html'),'-helpbrowser')
  Pressure_Drop_StorageHX : Subsystem  mask(Pressure drop of tube heat exchanger in a storage){dia=0.1, hgt=1, dplin=10, dpqua=10}
      mask prompts: dia "Diameter of HX pipe [m]"; hgt "Height difference inlet-outlet [m]"; dplin "Pressure drop coefficient dplin [Pa/(kg/s)]"; dpqua "Pressure drop coefficient dpqua [Pa/(kg/s)²]"
      mask help:
      | Calculates the pressure drop in a tube heat exchanger according to:
      | dp = dpqua*mdot^2 + dplin*mdot + density*grav*height
      | with grav = 9.18 kg*m/s²
      mask Help: web(fullfile(path_carnot('help'),'Pressure_Drop_StorageHX.html'),'-helpbrowser')
  Pressure_Drop_StoragePipe : Subsystem  mask(Pressure drop pipe connection of a storage){dpipe=0.04, dstg=1, hgt=2}
      mask prompts: dpipe "Diameter of pipe in m"; dstg "Diameter of storage in m"; hgt "Height difference inlet-outlet"
      mask help: Calculates the pressure drop in a pipe connection to a storage respecting the diameter changes and the static height difference. The temperature for the density is taken from the storage nodes.
      mask Help: web(fullfile(path_carnot('help'),'Pressure_Drop_StoragePipe.html'),'-helpbrowser')
      mask TypeOptions dpipe: Pressure_Drop_changeD/dia | Pressure_Drop_decreaseD/dia
      mask TypeOptions dstg: Pressure_Drop_increaseD/dia
      mask TypeOptions hgt: Constant/Value
  Pressure_Drop_changeD : Subsystem  mask(Pressure Drop Change Diameter){dia=1}
      mask prompts: dia "Diameter in m"
      mask help: Calculates the pressure drop due to a diameter change at the inlet (of a pipe).
      mask Help: web(fullfile(path_carnot('help'),'Pressure_Drop_changeD.html'),'-helpbrowser')
  Pressure_Drop_staticHeight : Subsystem  mask(Pressure Drop static Height){}
      mask help:
      | Pressure drop or increase due to statig height.
      | Calculation is done for ID > 20000 (dp = f(h)).
      | dp = height/Nnodes*grav*density(Tnodes)
      | The length of Tnodes defines the number of temperature nodes.
      | The height is between inlet and outlet. It is divided by the number of nodes Nnodes in the temperature vector "Tnodes".
      | Height is positive for outlet above inlet when pressure decreases.
      mask Help: web(fullfile(path_carnot('help'),'Pressure_Drop_staticHeight.html'),'-helpbrowser')
  Pressuredrop : Subsystem  mask(pressure drop){}
      mask help:
      | Pressure drop according to input values of con, lin and qua:
      | dp = con + lin*mdot + qua*mdot²
      | The coefficients are also added to the correponding THB elements.
      mask Help: web(fullfile(path_carnot('help'),'Pressuredrop.html'),'-helpbrowser')
  clq2friction_coeff : Subsystem  mask(clq 2 friction coefficient){Value=0.05, Gain=1}
      mask prompts: Value "Diameter of pipe in m"; Gain "Pipe length in m"
      mask help:
      | Determine the pipe friction coefficent lambda coefficient from clq:
      | dp = lambda * length * denstiy / (dia * 2) * v^2
      | for round pipes:
      | dp  = 8 * lambda * l * mdot^2 / (rho * pi^2 * dia^5)
      | Carnot pressure drop calculation:
      | dp = c + l*mdot + q*mdot^2
      | so:  lambda = q * rho * pi^2 * dia^5 / (8 * l)
      | c = 0; l = 0;
      | and l = 0; c = 0;
      mask TypeOptions Value: diameter/Value
      mask TypeOptions Gain: length/Gain
  clq2pressuredropcoeff : Subsystem  mask(pressure drop coefficient 2 clq){}
      mask help:
      | Calculate the clq coefficients from the pressure drop coefficients.
      | dp = zeta * density/2 * w^2
      | dp = c + l*mdot + q*mdot^2    Carnot approach (here c = l = 0)
      | with mdot = Vdot*density = w*A*density  -> w = mdot/A/density
      | dp = zeta * density/2 * mdot^2/A^2/density^2
      | dp = zeta/(2*A^2*density) * mdot^2
      | -> q = zeta/(2*A^2*density)
      | with A = pi/4*d^2
      | -> q = 8*zeta / (pi^2*d^4*density)
  friction_coeff2clq : Subsystem  mask(friction coefficient 2 clq){Value=0.05, Gain=1}
      mask prompts: Value "Diameter of pipe in m"; Gain "Pipe length in m"
      mask help:
      | Determine the clq coefficients from pipe friction coefficent lambda:
      | dp = lambda * length * denstiy / (dia * 2) * v^2
      | for round pipes:
      | dp  = 8 * lambda * l * mdot^2 / (rho * pi^2 * dia^5)
      | Carnot pressure drop calculation:
      | dp = c + l*mdot + q*mdot^2
      | so:  q = 8 * lambda * l / (rho * pi^2 * dia^5)
      | and l = 0; c = 0;
      mask TypeOptions Value: diameter/Value
      mask TypeOptions Gain: length/Gain
  pressuredropcoeff2clq : Subsystem  mask(pressure drop coefficient 2 clq){}
      mask help:
      | Calculate the clq coefficients from the pressure drop coefficients.
      | dp = zeta * density/2 * w^2
      | dp = c + l*mdot + q*mdot^2    Carnot approach (here c = l = 0)
      | with mdot = Vdot*density = w*A*density  -> w = mdot/A/density
      | dp = zeta * density/2 * mdot^2/A^2/density^2
      | dp = zeta/(2*A^2*density) * mdot^2
      | -> q = zeta/(2*A^2*density)
      | with A = pi/4*d^2
      | -> q = 8*zeta / (pi^2*d^4*density)
  relFlowCoeff2qua : Subsystem  mask{kvs=1.6}
      mask prompts: kvs "Flow coefficient of open valve (Kvs) in m³/h"
      mask TypeOptions kvs: Kvs/Gain
      mask Display: disp('rel\nFlow Coeff\nto qua')
